simulink model "simu2"  (R2024a)
settings: Solver=VariableStepAuto  StartTime=0.0  StopTime=10.0  RelTol=1e-3
settings Model: Creator=psp_dada  LastModifiedBy=psp_dada

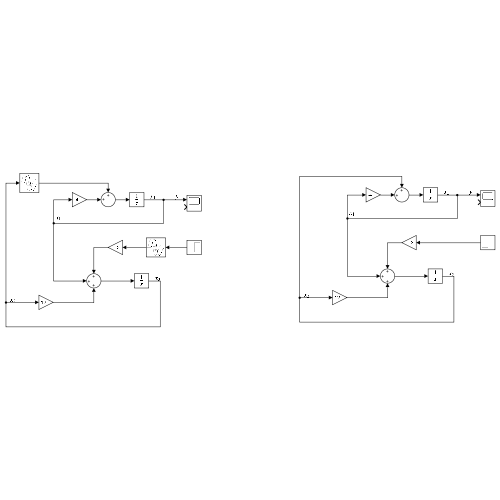
[thumbnail: Simulink's stored preview of the top-level diagram]
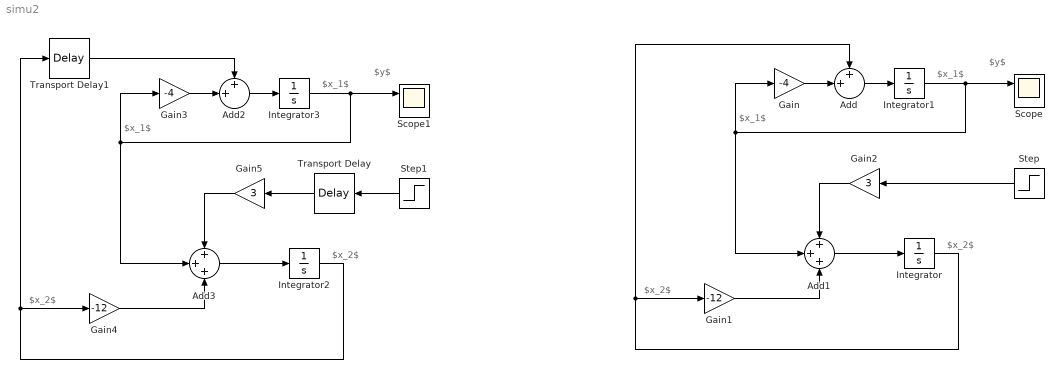
== system simu2 ==
  note: $x_2$
  note: $x_2$
  note: $x_1$
  note: $x_1$
  note: $y$
  note: $x_2$
  note: $y$
  note: $x_2$
  note: $x_1$
  note: $x_1$
  Add : Sum  Inputs=++|
  Add1 : Sum  Inputs=+++
  Add2 : Sum  Inputs=++|
  Add3 : Sum  Inputs=+++
  Gain : Gain  Gain=-4
  Gain1 : Gain  Gain=-12
  Gain2 : Gain  Gain=3
  Gain3 : Gain  Gain=-4
  Gain4 : Gain  Gain=-12
  Gain5 : Gain  Gain=3
  Integrator{,1..3} (4 alike) : Integrator
  Scope : Scope  NumInputPorts=2
  Scope1 : Scope  NumInputPorts=2
  Step : Step  SampleTime=0.001
  Step1 : Step  SampleTime=0.001
  Transport Delay : TransportDelay  DelayTime=0.2
  Transport Delay1 : TransportDelay  DelayTime=0.4
  wires:
  Add1/1 -> Integrator/1
  Gain2/1 -> Add1/1
  Gain1/1 -> Add1/3
  Integrator/1 -> Add/1, Gain1/1
  Gain/1 -> Add/2
  Add/1 -> Integrator1/1
  Integrator1/1 -> Add1/2, Gain/1, Scope/1
  Step/1 -> Gain2/1
  Gain5/1 -> Add3/1
  Gain4/1 -> Add3/3
  Add3/1 -> Integrator2/1
  Gain3/1 -> Add2/2
  Add2/1 -> Integrator3/1
  Integrator3/1 -> Add3/2, Gain3/1, Scope1/1
  Integrator2/1 -> Transport Delay1/1, Gain4/1
  Step1/1 -> Transport Delay/1
  Transport Delay/1 -> Gain5/1
  Transport Delay1/1 -> Add2/1
